simulink model "sgMdl_IO324_AnalogLoopback"  (R2024b)
settings: Solver=FixedStepAuto  StartTime=0.0  StopTime=inf  RelTol=1e-3
undefined symbols (not defined in the file): Ended, IO3xx, Pull, pull, Single, up
libraries: speedgoatlib_fpga_analog_io x3, slrealtimeloglib x2, simulink x1, speedgoatlib_fpga x1
Description:
  | IO324 - Analog Loopback
settings Model: ModifiedByFormat=Speedgoat  SimulationMode=external  ExtModeTrigDuration=100000  Creator=Speedgoat  LastModifiedBy=Speedgoat
settings SolverCC: ConcurrentTasks=on  PositivePriorityOrder=on
settings DataIOCC: SaveFormat=StructureWithTime
settings OptimizationCC: BlockReduction=off  OptimizeBlockIOStorage=off  BufferReuse=off  ReuseModelBlockBuffer=off
settings DebuggingCC: UnderspecifiedInitializationDetection=Classic  MergeDetectMultiDrivingBlocksExec=none  TasksWithSamePriorityMsg=none
settings HardwareCC: ProdBitPerLong=64  ProdLongLongMode=on  ProdHWDeviceType=Intel->x86-64 (Linux 64)
settings ModelReferenceCC: EnableRefExpFcnMdlSchedulingChecks=on  PropagateSignalLabelsOutOfModel=off
settings RTWCC: Description=Speedgoat Real-Time Target Machine  SystemTargetFile=speedgoat.tlc  TemplateMakefile=slrealtime_default_tmf  PostCodeGenCommand=sg.model.build.makeCfg(bdroot, buildInfo);  Toolchain=Simulink Real-Time Toolchain  BuildConfiguration=Faster Runs  TargetLang=C++  GPUComputeCapability=3.5
settings SimulinkRealTimeTargetCC: SubcomponentCodeInterfacePackaging=Reusable function  InstructionSetFMA=off  LogToMDFFile=off  SLRTFileLogMaxRuns=10
settings ConfigComp: CovBoundaryAbsTol=1.0e-5

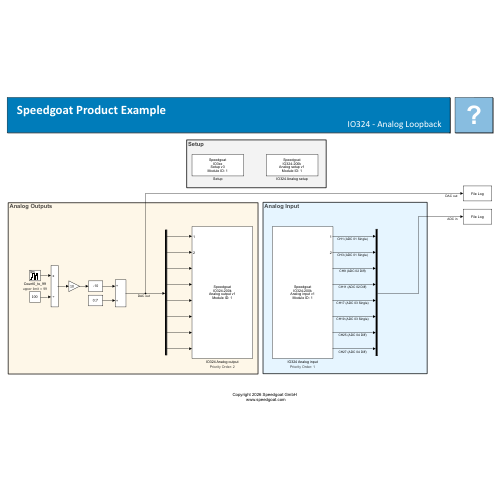
[thumbnail: Simulink's stored preview of the top-level diagram]
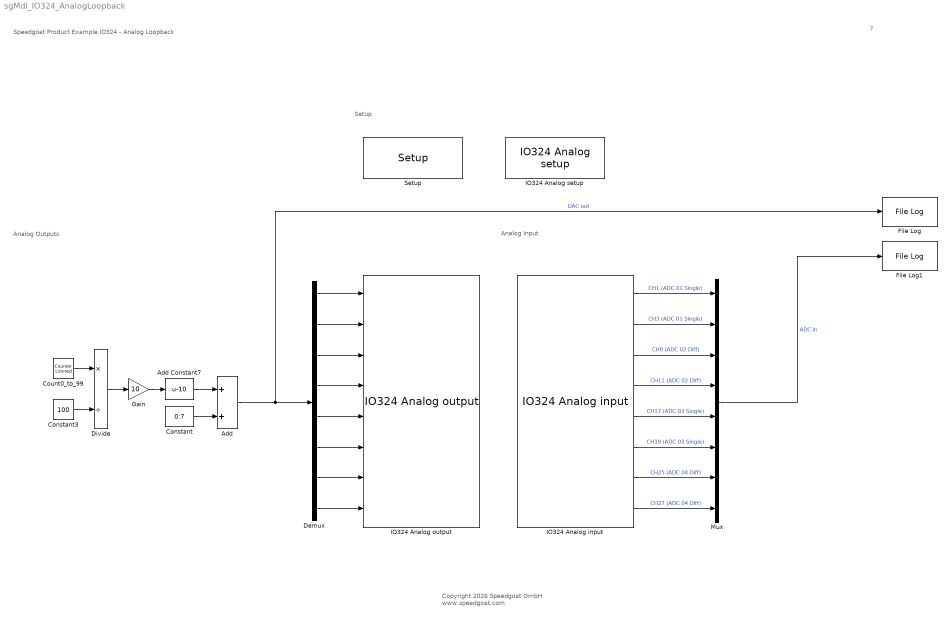
== system sgMdl_IO324_AnalogLoopback ==
  note: Analog Outputs
  note: Analog Input
  note: Setup
  note: Speedgoat Product Example
      | IO324 - Analog Loopback
  note: ?
  note: Copyright 2026 Speedgoat GmbH
      |  www.speedgoat.com
  Add : Sum
  Add Constant7 : Bias  Bias=-10  SaturateOnIntegerOverflow=off
  Constant : Constant  Value=0:7  SampleTime=-1
  Constant3 : Constant  Value=100  SampleTime=-1
  Count0_to_99 : simulink/Sources/Counter Limited  uplimit=99  tsamp=-1
      settings: AttributesFormatString=upper limit = %<uplimit>
  Demux : Demux  Outputs=8
  Divide : Product  Inputs=*/
  File Log : slrealtimeloglib/File Log  decimation=1  inputProcessing=Elements as channels (sample based)
  File Log1 : slrealtimeloglib/File Log  decimation=1  inputProcessing=Elements as channels (sample based)
  Gain : Gain  Gain=10
  IO324 Analog input : speedgoatlib_fpga_analog_io/IO324/IO324 Analog input  Priority=1  id=1  parSampleTime=-1  parPciSlot=-1  parAiChannels=[1 3 9 11 17 19 25 27]  parAiTriggerMode=[1 1 1 1]  parAiReadPrevValue=0  parAiEnableFrame=0  parAiVoltageRange=[2 2 2 2 2 2 2 2]  parAdcCoupling=[1 1 1 1]  parAdcContSampling=0  parAdcDmaEnable=0  parAdcActiveDmaDevices=[1 1 1 1]  parAiFrameSize=-1
      settings: AttributesFormatString=Priority Order: %<Priority>  SourceProductName=Simulink Real-Time: Speedgoat I/O Blockset
  IO324 Analog output : speedgoatlib_fpga_analog_io/IO324/IO324 Analog output  Priority=2  id=1  parSampleTime=-1  parPciSlot=-1  parAoChannels=[1 2 3 4 5 6 7 8]  parAoVoltageRange=[1 1 1 1 1 1 1 1]  parDacOverRange=[0 0 0 0 0 0 0 0]  parAoInitValues=[-10 -9 -8 -7 -6 -5 -4 -3]  parAoReset=[1 0 1 0 1 0 1 0]  parDacSyncOut=1  parAoEnableFrame=0  parDacActiveDmaDevices=[1 1 1 1]  parDacDmaLatency=2  parAoFrameSize=100
      settings: AttributesFormatString=Priority Order: %<Priority>  SourceProductName=Simulink Real-Time: Speedgoat I/O Blockset
  IO324 Analog setup : speedgoatlib_fpga_analog_io/IO324/IO324 Analog setup  id=1  parEnableCodeModule1=off  parEnableCodeModule2=off  parEnableCodeModule3=off  parEnableCodeModule4=off  parEnableCodeModule5=off  parEnableCodeModule6=off  parEnableCodeModule7=off  parEnableCodeModule8=off  parAdcEnableIndividualTrigger=off  parAdcTriggerMode1=Model Step  parAdcSampleRate1=100e3  parAdcDioTriggerChannel1=1  parAdcInternalTrigger1=<empty>  parAdcOversampling1=None  parAdcTriggerMode2=Model Step  parAdcSampleRate2=100e3  parAdcDioTriggerChannel2=1  parAdcInternalTrigger2=<empty>  parAdcOversampling2=None  parAdcTriggerMode3=Model Step  parAdcSampleRate3=100e3  parAdcDioTriggerChannel3=1  parAdcInternalTrigger3=<empty>  parAdcOversampling3=None  parAdcTriggerMode4=Model Step  parAdcSampleRate4=100e3  parAdcDioTriggerChannel4=1  parAdcInternalTrigger4=<empty>  parAdcOversampling4=None  parAdcReadPrevValueIndividualTrigger=on  parAdcEnableFrame=off  parAdcTriggerMode=Model Step  parAdcReadPrevValue=off  parAdcSampleRate=100e3  parAdcDioTriggerChannel=1  parAdcInternalTrigger=<empty>  parAdcOversampling=None  parAdcTriggerResolution=1e-08  parAdcSampleRateFrame=100e3  parAdcFrameSize=-1  parAdcSampleTime=1e-3  parDacTriggerMode=Model Step  parDacInternalTrigger=<empty>  parDacDioTriggerChannel=0  parDacEnableFrame=off  dacUsesTimer=off  parDacFifoThreshold=100  parDacTriggerResolution=1e-08  parDacSampleRate=5e6  parDacFrameSize=100  parDacSampleTime=-1  parAdcCoupling1=Single-Ended  parAdcChannel1=on  parAdcChannel2=off  parAdcChannel3=on  parAdcChannel4=off  parAdcChannel5=off  parAdcChannel6=off  parAdcChannel7=off  parAdcChannel8=off  parAdcRangeAll1=+-10.24 V  parVoltageRangePerChannelEn1=off  parAdcRange1=+-10.24 V  parAdcRange5=+-10.24 V  parAdcRange2=+-10.24 V  parAdcRange6=+-10.24 V  parAdcRange3=+-10.24 V  parAdcRange7=+-10.24 V  parAdcRange4=+-10.24 V  parAdcRange8=+-10.24 V  parAdcCoupling2=Differential  parAdcChannel9=on  parAdcChannel10=on  parAdcChannel11=on  parAdcChannel12=off  parAdcChannel13=off  parAdcChannel14=off  parAdcChannel15=off  parAdcChannel16=off  parAdcRangeAll2=+-10.24 V  parVoltageRangePerChannelEn2=off  parAdcRange9=+-10.24 V  parAdcRange13=+-10.24 V  parAdcRange10=+-10.24 V  parAdcRange14=+-10.24 V  parAdcRange11=+-10.24 V  parAdcRange15=+-10.24 V  parAdcRange12=+-10.24 V  parAdcRange16=+-10.24 V  parAdcCoupling3=Single-Ended  parAdcChannel17=on  parAdcChannel18=off  parAdcChannel19=on  parAdcChannel20=off  parAdcChannel21=off  parAdcChannel22=off  parAdcChannel23=off  parAdcChannel24=off  parAdcRangeAll3=+-10.24 V  parVoltageRangePerChannelEn3=off  parAdcRange17=+-10.24 V  parAdcRange21=+-10.24 V  parAdcRange18=+-10.24 V  parAdcRange22=+-10.24 V  parAdcRange19=+-10.24 V  parAdcRange23=+-10.24 V  parAdcRange20=+-10.24 V  parAdcRange24=+-10.24 V  parAdcCoupling4=Differential  parAdcChannel25=on  parAdcChannel26=on  parAdcChannel27=on  parAdcChannel28=off  parAdcChannel29=off  parAdcChannel30=off  parAdcChannel31=off  parAdcChannel32=off  parAdcRangeAll4=+-10.24 V  parVoltageRangePerChannelEn4=off  parAdcRange25=+-10.24 V  parAdcRange29=+-10.24 V  parAdcRange26=+-10.24 V  parAdcRange30=+-10.24 V  parAdcRange27=+-10.24 V  parAdcRange31=+-10.24 V  parAdcRange28=+-10.24 V  parAdcRange32=+-10.24 V  parAdcAutoCorrection=on  parDacChannel1=on  parDacChannel2=on  parDacChannel3=on  parDacChannel4=on  parDacChannel5=on  parDacChannel6=on  parDacChannel7=on  parDacChannel8=on  parDacRange1=+-10 V  parDacInitValue1=-10  parDacReset1=on  parDacRange2=+-10 V  parDacInitValue2=-9  parDacReset2=off  parDacRange3=+-10 V  parDacInitValue3=-8  parDacReset3=on  parDacRange4=+-10 V  parDacInitValue4=-7  parDacReset4=off  parDacRange5=+-10 V  parDacInitValue5=-6  parDacReset5=on  parDacRange6=+-10 V  parDacInitValue6=-5  parDacReset6=off  parDacRange7=+-10 V  parDacInitValue7=-4  parDacReset7=on  parDacRange8=+-10 V  parDacInitValue8=-3  parDacReset8=off  parDacAutoCorrection=on
      settings: SourceProductName=Simulink Real-Time: Speedgoat I/O Blockset
  Mux : Mux  Inputs=8
  Setup : speedgoatlib_fpga/Setup/Setup  board=Please select...  id=1  pciSlot=-1  device_id=1  bitstreamFilePath=C:\Work\SVN\Speedgoatlib\releases\10.0.0\product_examples\IO324\IO324_helper\  bitstreamFile=Please select...  fpgaFreq=[100000000 100000000]  enableDma=on  rearEnb_1=off  rearIO_1=IO3xx-21  rearEnb_2=off  rearIO_2=None  ProgSpiFlash=off  ProgBPIFlash=off  useFpgaDmaController=off  dmaTrigDropdown=Model Step  dmaTrigSelect=0  dmaStopOnOverload=on  dmaModeSequential=on  dmaModeParallel=off  PullRPort15=pull-up 3.3V  PullRPort31=pull-up 3.3V  PullRPort47=pull-up 3.3V  PullRPort63=pull-up 3.3V  diffLineTermination_1=on  diffLineTermination_2=on  diffLineTermination_3=on  diffLineTermination_4=on  diffLineTermination_5=on  diffLineTermination_6=on  diffLineTermination_7=on  diffLineTermination_8=on  diffLineTermination_9=on  diffLineTermination_10=on  diffLineTermination_11=on  diffLineTermination_12=on  diffLineTermination_13=on  diffLineTermination_14=on  diffLineTermination_15=on  diffLineTermination_16=on  diffLineTermination_17=on  diffLineTermination_18=on  diffLineTermination_19=on  diffLineTermination_20=on  diffLineTermination_21=on  diffLineTermination_22=on  diffLineTermination_23=on  diffLineTermination_24=on  diffLineTermination_25=on  diffLineTermination_26=on  diffLineTermination_27=on  diffLineTermination_28=on  diffLineTermination_29=on  diffLineTermination_30=on  diffLineTermination_31=on  diffLineTermination_32=on  ioVoltageDropDown1=3.3V  pullResistorDropDown1_1=Pull-up  pullResistorDropDown1_2=Pull-up  pullResistorDropDown1_3=Pull-up  pullResistorDropDown1_4=Pull-up  pullResistorDropDown1_5=Pull-up  pullResistorDropDown1_6=Pull-up  pullResistorDropDown1_7=Pull-up  pullResistorDropDown1_8=Pull-up  ttlIsImplementedCheckBox1=off  pullResistorDropDown2=Pull-up  ioVoltageDropDown2=3.3V  ttlIsImplementedCheckBox2=off  pullResistorDropDown3=Pull-up  ioVoltageDropDown3=3.3V  ttlIsImplementedCheckBox3=off  pullResistorDropDown4=Pull-up  ioVoltageDropDown4=3.3V  ttlIsImplementedCheckBox4=off  pullResistorDropDown5=Pull-up  ioVoltageDropDown5=3.3V  ttlIsImplementedCheckBox5=off  pullResistorDropDown6=Pull-up  ioVoltageDropDown6=3.3V  ttlIsImplementedCheckBox6=off  pullResistorDropDown7=Pull-up  ioVoltageDropDown7=3.3V  ttlIsImplementedCheckBox7=off  pullResistorDropDown8=Pull-up  ioVoltageDropDown8=3.3V  ttlIsImplementedCheckBox8=off  terminationCheckBox1=off  terminationCheckBox2=off  terminationCheckBox3=off  terminationCheckBox4=off  diffIsImplementedCheckBox1=off  terminationCheckBox5=off  terminationCheckBox6=off  terminationCheckBox7=off  terminationCheckBox8=off  diffIsImplementedCheckBox2=off  terminationCheckBox9=off  terminationCheckBox10=off  terminationCheckBox11=off  terminationCheckBox12=off  diffIsImplementedCheckBox3=off  terminationCheckBox13=off  terminationCheckBox14=off  terminationCheckBox15=off  terminationCheckBox16=off  diffIsImplementedCheckBox4=off  terminationCheckBox17=off  terminationCheckBox18=off  terminationCheckBox19=off  terminationCheckBox20=off  diffIsImplementedCheckBox5=off  terminationCheckBox21=off  terminationCheckBox22=off  terminationCheckBox23=off  terminationCheckBox24=off  diffIsImplementedCheckBox6=off  terminationCheckBox25=off  terminationCheckBox26=off  terminationCheckBox27=off  terminationCheckBox28=off  diffIsImplementedCheckBox7=off  terminationCheckBox29=off  terminationCheckBox30=off  terminationCheckBox31=off  terminationCheckBox32=off  diffIsImplementedCheckBox8=off  PullRPort0_1=pull-up  VioPort0_1=3.3V  PullRPort1_1=pull-up  VioPort1_1=3.3V  PullRPort2_1=pull-up  VioPort2_1=3.3V  PullRPort3_1=pull-up  VioPort3_1=3.3V  PullRPort4_1=pull-up  VioPort4_1=3.3V  PullRPort5_1=pull-up  VioPort5_1=3.3V  PullRPort6_1=pull-up  VioPort6_1=3.3V  diffLineTermination_rear1_1=on  diffLineTermination_rear1_2=on  diffLineTermination_rear1_3=on  diffLineTermination_rear1_4=on  diffLineTermination_rear1_5=on  diffLineTermination_rear1_6=on  diffLineTermination_rear1_7=on  diffLineTermination_rear1_8=on  PullRPort0_2=pull-up  VioPort0_2=3.3V  PullRPort1_2=pull-up  VioPort1_2=3.3V  PullRPort2_2=pull-up  VioPort2_2=3.3V  PullRPort3_2=pull-up  VioPort3_2=3.3V  PullRPort4_2=pull-up  VioPort4_2=3.3V  PullRPort5_2=pull-up  VioPort5_2=3.3V  PullRPort6_2=pull-up  VioPort6_2=3.3V  diffLineTermination_rear2_1=on  diffLineTermination_rear2_2=on  diffLineTermination_rear2_3=on  diffLineTermination_rear2_4=on  diffLineTermination_rear2_5=on  diffLineTermination_rear2_6=on  diffLineTermination_rear2_7=on  diffLineTermination_rear2_8=on
      settings: SourceProductName=IO3xx
  wires:
  Divide/1 -> Gain/1
  Constant3/1 -> Divide/2
  Count0_to_99/1 -> Divide/1
  Gain/1 -> Add Constant7/1
  Add Constant7/1 -> Add/1
  Demux/3 -> IO324 Analog output/3
  Demux/5 -> IO324 Analog output/5
  Demux/4 -> IO324 Analog output/4
  Demux/8 -> IO324 Analog output/8
  Demux/6 -> IO324 Analog output/6
  Demux/7 -> IO324 Analog output/7
  Demux/1 -> IO324 Analog output/1
  Demux/2 -> IO324 Analog output/2
  Constant/1 -> Add/2
  IO324 Analog input/2 -> Mux/2  "CH3 (ADC 01 Single)"
  IO324 Analog input/3 -> Mux/3  "CH9 (ADC 02 Diff)"
  IO324 Analog input/1 -> Mux/1  "CH1 (ADC 01 Single)"
  IO324 Analog input/4 -> Mux/4  "CH11 (ADC 02 Diff)"
  IO324 Analog input/5 -> Mux/5  "CH17 (ADC 03 Single)"
  IO324 Analog input/6 -> Mux/6  "CH19 (ADC 03 Single)"
  IO324 Analog input/7 -> Mux/7  "CH25 (ADC 04 Diff)"
  IO324 Analog input/8 -> Mux/8  "CH27 (ADC 04 Diff)"
  Add/1 -> File Log/1, Demux/1  "DAC out"
  Mux/1 -> File Log1/1  "ADC in"
